simulink model "qhug_5"  (R2017a)
settings: Solver=ode4  StartTime=0.0  StopTime=3000  FixedStep=0.1  MaxStep=0.01  RelTol=1e-3
settings Model: Creator=daoist  LastModifiedBy=daoist
settings DataIOCC: ReturnWorkspaceOutputs=on
settings DebuggingCC: SFMachineParentedDataDiag=error
settings SFSimCC: SimUseLocalCustomCode=on
settings RTWCC: RTWUseLocalCustomCode=on

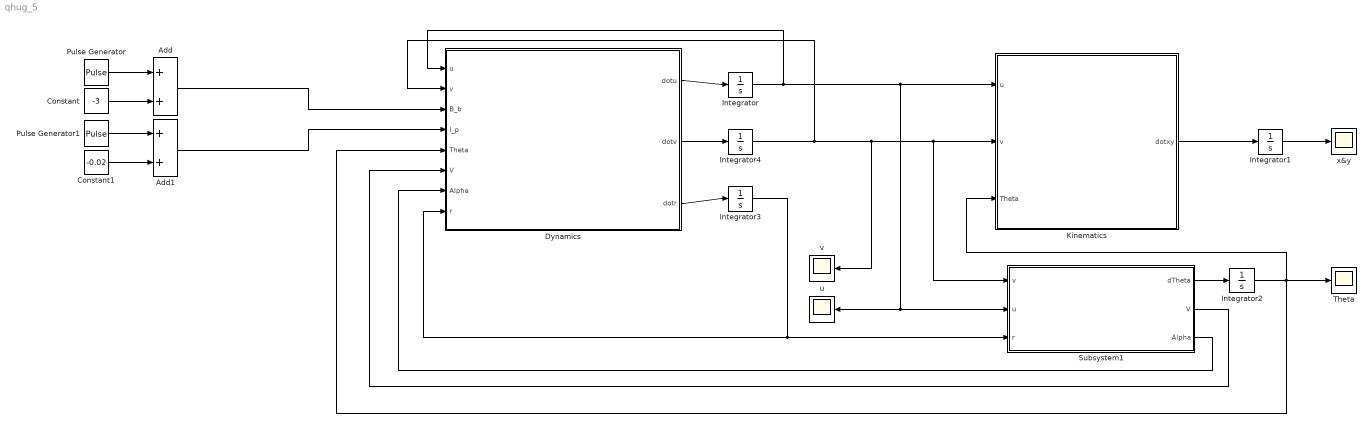
== system qhug_5 ==
  Add : Sum
  Add1 : Sum
  Constant : Constant  Value=-3
  Constant1 : Constant  Value=-0.02
  Dynamics : Subsystem
  Integrator : Integrator  InitialCondition=0.01  UpperSaturationLimit=[inf 0.05]  LowerSaturationLimit=-[inf 0.05]
  Integrator1 : Integrator
  Integrator2 : Integrator
  Integrator3 : Integrator
  Integrator4 : Integrator  UpperSaturationLimit=[ 0.05]  LowerSaturationLimit=-[ 0.05]
  Kinematics : Subsystem
  Pulse Generator : DiscretePulseGenerator  PulseType=Time based  Amplitude=6  Period=1500  PulseWidth=50  PhaseDelay=750
  Pulse Generator1 : DiscretePulseGenerator  PulseType=Time based  Amplitude=0.04  Period=1500  PulseWidth=50
  Subsystem1 : Subsystem
  Theta : Scope
  u : Scope
  v : Scope
  x&y : Scope
  wires:
  Dynamics/1(dotu) -> Integrator/1
  Integrator/1 -> Kinematics/1(u), Subsystem1/2(u), u/1, Dynamics/1(u)
  Kinematics/1(dotxy) -> Integrator1/1
  Integrator1/1 -> x&y/1
  Subsystem1/1(dTheta) -> Integrator2/1
  Dynamics/3(dotr) -> Integrator3/1
  Integrator3/1 -> Subsystem1/3(r), Dynamics/8(r)
  Pulse Generator1/1 -> Add1/1
  Add/1 -> Dynamics/3(B_b)
  Constant/1 -> Add/2
  Add1/1 -> Dynamics/4(l_p)
  Constant1/1 -> Add1/2
  Pulse Generator/1 -> Add/1
  Subsystem1/2(V) -> Dynamics/6(V)
  Integrator2/1 -> Theta/1, Dynamics/5(Theta), Kinematics/3(Theta)
  Subsystem1/3(Alpha) -> Dynamics/7(Alpha)
  Dynamics/2(dotv) -> Integrator4/1
  Integrator4/1 -> Kinematics/2(v), Subsystem1/1(v), v/1, Dynamics/2(v)

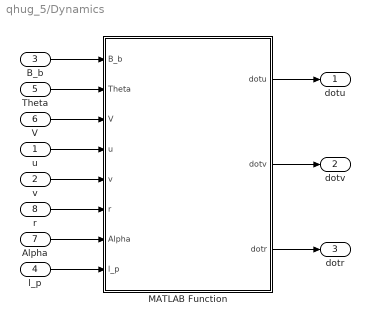
== system qhug_5/Dynamics ==
  u : Inport
  v : Inport  Port=2
  B_b : Inport  Port=3
  l_p : Inport  Port=4
  Theta : Inport  Port=5
  V : Inport  Port=6
  Alpha : Inport  Port=7
  r : Inport  Port=8
  MATLAB Function : MATLAB Function  TreatAsAtomicUnit=on
  dotu : Outport
  dotv : Outport  Port=2
  dotr : Outport  Port=3
  wires:
  v/1 -> MATLAB Function/5(v)
  MATLAB Function/2(dotv) -> dotv/1
  MATLAB Function/3(dotr) -> dotr/1
  B_b/1 -> MATLAB Function/1(B_b)
  Theta/1 -> MATLAB Function/2(Theta)
  V/1 -> MATLAB Function/3(V)
  r/1 -> MATLAB Function/6(r)
  Alpha/1 -> MATLAB Function/7(Alpha)
  l_p/1 -> MATLAB Function/8(l_p)
  u/1 -> MATLAB Function/4(u)
  MATLAB Function/1(dotu) -> dotu/1

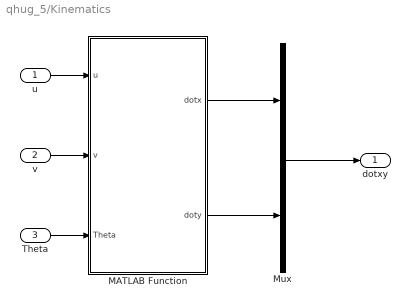
== system qhug_5/Kinematics ==
  u : Inport
  v : Inport  Port=2
  Theta : Inport  Port=3
  MATLAB Function : MATLAB Function  TreatAsAtomicUnit=on
  Mux : Mux  Inputs=2
  dotxy : Outport
  wires:
  v/1 -> MATLAB Function/2(v)
  u/1 -> MATLAB Function/1(u)
  MATLAB Function/1(dotx) -> Mux/1
  MATLAB Function/2(doty) -> Mux/2
  Mux/1 -> dotxy/1
  Theta/1 -> MATLAB Function/3(Theta)

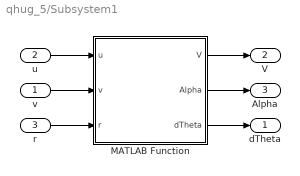
== system qhug_5/Subsystem1 ==
  v : Inport
  u : Inport  Port=2
  r : Inport  Port=3
  MATLAB Function : MATLAB Function  TreatAsAtomicUnit=on
  dTheta : Outport
  V : Outport  Port=2
  Alpha : Outport  Port=3
  wires:
  v/1 -> MATLAB Function/2(v)
  r/1 -> MATLAB Function/3(r)
  MATLAB Function/2(Alpha) -> Alpha/1
  MATLAB Function/3(dTheta) -> dTheta/1
  MATLAB Function/1(V) -> V/1
  u/1 -> MATLAB Function/1(u)

== matlab function qhug_5/Subsystem1/MATLAB Function ==
  data: u input; V output; v input; Alpha output; r input; dTheta output
function [V,Alpha, dTheta] = VV(u,v, r)

V = sqrt(u^2 + v^2);
Alpha = -atan(v/u);
dTheta = r;

== matlab function qhug_5/Kinematics/MATLAB Function ==
  data: u input; dotx output; doty output; v input; Theta input
function [dotx,doty] = VK(u,v, Theta)

dotx = u * cos(Theta) - v * sin(Theta);
doty = u * sin(Theta) + v * sin(Theta);

== matlab function qhug_5/Dynamics/MATLAB Function ==
  data: B_b input; Theta input; V input; u input; dotu output; v input; r input; Alpha input; l_p input; dotv output; dotr output
function [dotu,dotv,dotr] = VD(B_b, Theta, V, u, v, r,  Alpha, l_p)
m = 69;
m_p = 18;
m_r = 18;
rho = 1022;
B_0 = 676.2;
g = 9.8;
lambda_11 = 2;
lambda_22 = 75.8;
lambda_33 = 102.9;
lambda_44 = 9.5;
lambda_55 = 43;
lambda_66 = 31;
lambda_26 = -12;
lambda_35 = 33;
J_Bx = 0.55;
J_By = 22.36;
J_Bz = 22.3;

y_G = 0.0047;

A_D = 0.038;
L = 2.17;
l_b = 0.93;
t = 0.16;
K_T = 0.34;
K_Q = 0.067;
d_p = 0.12;
C_x = -0.42;
C_ay = 0.316;
C_ry = -8.37;

T_az = -0.0573;
T_rz = -2.34;

r1 = r * L / V;

G = g * m;

A=[ m + lambda_11 , 0 , -m * y_G;
    0, m + lambda_22, lambda_26;
    m*y_G, lambda_26, J_Bz + lambda_66
    ];
B = [-B_b * sin(Theta) ...
    + ( G - B_0) * sin(Theta) ...
    + 0.5 * rho * V^2 * A_D * C_x ...
    + m * v * r ... ,
    -B_b * cos(Theta) ...
    + ( G - B_0) * cos(Theta) ...
    + 0.5 * rho * V^2 * A_D * (C_ay * Alpha + C_ry * r1) ...
    + m * y_G * r^2 ...
    - m * u * r ...,
    (B_b * l_b + m_p * g * l_p) * cos(Theta) ...
    + G * y_G * sin(Theta) ...
    + 0.5 * rho * V^2 * A_D * L * (T_az * Alpha + T_rz * r1) ...
    + m * y_G *  v * r ; ];
out = A \ B';
dotu = out(1);
dotv = out(2);
dotr = out(3);
